simulink model "tanques"  (R2018a)
settings: Solver=VariableStepAuto  StartTime=0.0  StopTime=10.0  RelTol=1e-3
undefined symbols (not defined in the file or in its folder): C2, R1, R1C1, R2
settings Model: Creator=carma  LastModifiedBy=carma

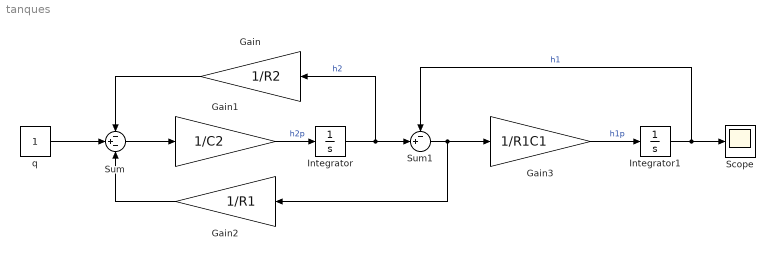
== system tanques ==
  Gain : Gain  Gain=1/R2
  Gain1 : Gain  Gain=1/C2
  Gain2 : Gain  Gain=1/R1
  Gain3 : Gain  Gain=1/R1C1
  Integrator : Integrator
  Integrator1 : Integrator
  Scope : Scope
  Sum : Sum  Inputs=-+-
  Sum1 : Sum  Inputs=-+|
  q : Constant
  wires:
  Gain/1 -> Sum/1
  Sum/1 -> Gain1/1
  Gain1/1 -> Integrator/1  "h2p"
  Integrator/1 -> Gain/1, Sum1/2  "h2"
  Gain2/1 -> Sum/3
  Sum1/1 -> Gain2/1, Gain3/1
  Gain3/1 -> Integrator1/1  "h1p"
  Integrator1/1 -> Sum1/1, Scope/1  "h1"
  q/1 -> Sum/2
